simulink model "flexible_drive_filtered"  (R2022a)
settings: Solver=ode45  StartTime=0.0  StopTime=2  RelTol=1e-3  EnableMultiTasking=on
values from neighbouring files (symbols this model uses):
  b1 = 0.0097    [q1_2.m]
  b2 = 0.00097122    [q1_2.m]
  d1 = 0.793    [q1_2.m]
  d2 = 0.0793    [q1_2.m]
  k = 0.0466    [q1_2.m]
  m1 = 0.00031218    [q1_2.m]
  m2 = 0.00016858    [q1_2.m]
undefined symbols (not defined in the file or in its folder): c, kp, q, sgn, Ts
settings Model: Creator=user  LastModifiedBy=mluser
settings SolverCC: AlgebraicLoopSolver=TrustRegion
settings DataIOCC: LimitDataPoints=on  SaveFormat=Array  SignalLoggingSaveFormat=ModelDataLogs  ReturnWorkspaceOutputs=off  SignalLoggingName=sigsOut
settings OptimizationCC: LifeSpan=inf
settings DebuggingCC: SaveWithParameterizedLinksMsg=none  UnderspecifiedInitializationDetection=Classic  MergeDetectMultiDrivingBlocksExec=none  SignalResolutionControl=TryResolveAllWithWarning  MultiTaskDSMMsg=warning  MultiTaskCondExecSysMsg=none  UnconnectedInputMsg=warning  UnconnectedOutputMsg=warning  UnconnectedLineMsg=warning  SFUnexpectedBacktrackingDiag=warning  SFNoUnconditionalDefaultTransitionDiag=warning  SFMachineParentedDataDiag=warning  ArithmeticOperatorsInVariantConditions=warning
settings HardwareCC: ProdBitPerPointer=32  ProdBitPerSizeT=32  ProdBitPerPtrDiffT=32  ProdLargestAtomicFloat=None  ProdIntDivRoundTo=Undefined  ProdEndianess=Unspecified  ProdWordSize=32  ProdHWDeviceType=32-bit Generic  TargetUnknown=on
settings ModelReferenceCC: PropagateSignalLabelsOutOfModel=off
settings SFSimCC: SimUseLocalCustomCode=off  CustomCodeUndefinedFunction=UseInterfaceOnly
settings RTWCC: RTWUseLocalCustomCode=off
settings CodeAppCC: StateflowObjectComments=on
settings GRTTargetCC: TargetLangStandard=C89/C90 (ANSI)  CombineOutputUpdateFcns=off  GRTInterface=on
settings ConfigComp: CovMetricSettings=dw  CovSaveCumulativeToWorkspaceVar=on  CovSaveSingleToWorkspaceVar=on  CovExternalEMLEnable=off

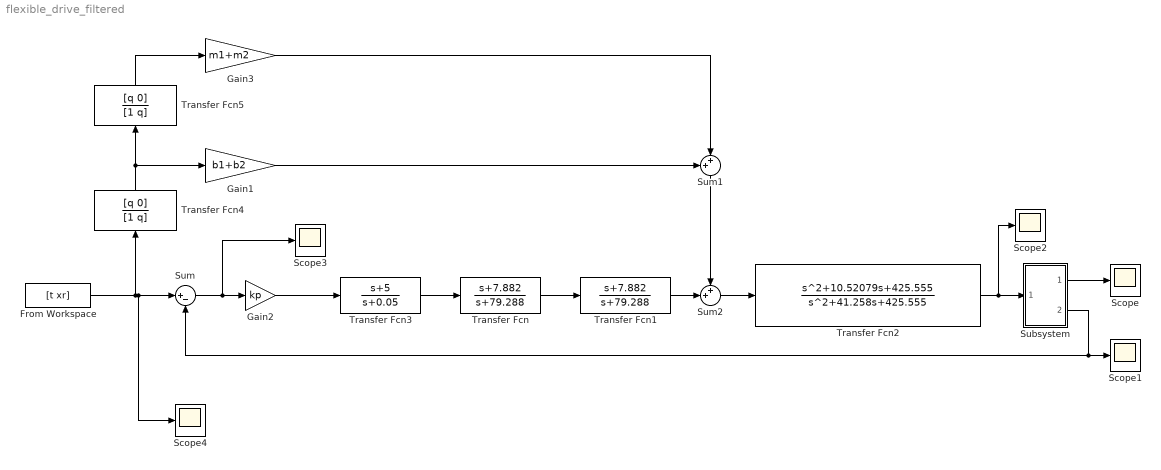
== system flexible_drive_filtered ==
  From Workspace : FromWorkspace  VariableName=[t xr]  SampleTime=Ts  ZeroCross=off  OutputAfterFinalValue=Holding final value
  Gain1 : Gain  Gain=b1+b2
  Gain2 : Gain  Gain=kp
  Gain3 : Gain  Gain=m1+m2
  Scope{,1..4} (5 alike) : Scope
  Subsystem : Subsystem
  Sum : Sum  Inputs=|+-
  Sum1 : Sum  Inputs=++|
  Sum2 : Sum  Inputs=++|
  Transfer Fcn : TransferFcn  Numerator=[1 7.882]  Denominator=[1 79.288]
  Transfer Fcn1 : TransferFcn  Numerator=[1 7.882]  Denominator=[1 79.288]
  Transfer Fcn2 : TransferFcn  Numerator=[1 10.52079 425.555]  Denominator=[1 41.258 425.555]
  Transfer Fcn3 : TransferFcn  Numerator=[1 5]  Denominator=[1 0.05]
  Transfer Fcn4 : TransferFcn  Numerator=[q 0]  Denominator=[1 q]
  Transfer Fcn5 : TransferFcn  Numerator=[q 0]  Denominator=[1 q]
  wires:
  From Workspace/1 -> Sum/1, Scope4/1, Transfer Fcn4/1
  Transfer Fcn2/1 -> Scope2/1, Subsystem/1(In1)
  Subsystem/1(Out1) -> Scope/1
  Subsystem/2(Out2) -> Scope1/1, Sum/2
  Transfer Fcn/1 -> Transfer Fcn1/1
  Sum/1 -> Scope3/1, Gain2/1
  Gain2/1 -> Transfer Fcn3/1
  Transfer Fcn3/1 -> Transfer Fcn/1
  Transfer Fcn4/1 -> Gain1/1, Transfer Fcn5/1
  Transfer Fcn5/1 -> Gain3/1
  Sum2/1 -> Transfer Fcn2/1
  Gain3/1 -> Sum1/2
  Gain1/1 -> Sum1/1
  Transfer Fcn1/1 -> Sum2/2
  Sum1/1 -> Sum2/1

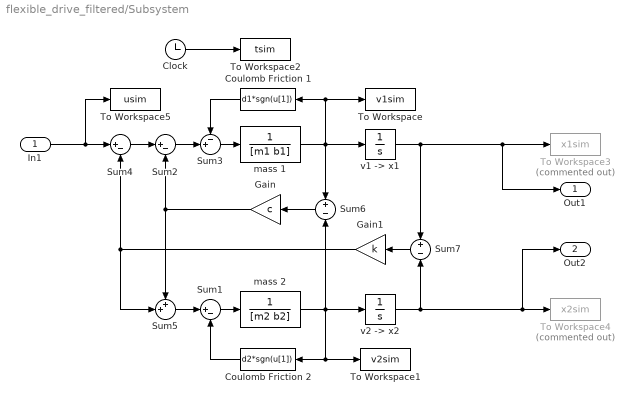
== system flexible_drive_filtered/Subsystem ==
  In1 : Inport
  Clock : Clock
  Coulomb Friction 1 : Fcn  Expr=d1*sgn(u[1])
  Coulomb Friction 2 : Fcn  Expr=d2*sgn(u[1])
  Gain : Gain  Gain=c  SaturateOnIntegerOverflow=on  OutDataTypeStr=Inherit: Same as input  ParamDataTypeStr=Inherit: Same as input
  Gain1 : Gain  Gain=k  SaturateOnIntegerOverflow=on  OutDataTypeStr=Inherit: Same as input  ParamDataTypeStr=Inherit: Same as input
  Sum1 : Sum  Inputs=|+-  SaturateOnIntegerOverflow=on
  Sum2 : Sum  Inputs=|+-  SaturateOnIntegerOverflow=on
  Sum3 : Sum  Inputs=-+|  SaturateOnIntegerOverflow=on
  Sum4 : Sum  Inputs=|+-  SaturateOnIntegerOverflow=on
  Sum5 : Sum  Inputs=++|  SaturateOnIntegerOverflow=on
  Sum6 : Sum  Inputs=+|-  SaturateOnIntegerOverflow=on
  Sum7 : Sum  Inputs=+|-  SaturateOnIntegerOverflow=on
  To Workspace : ToWorkspace  VariableName=v1sim  SampleTime=Ts
  To Workspace1 : ToWorkspace  VariableName=v2sim  SampleTime=Ts
  To Workspace2 : ToWorkspace  VariableName=tsim  SampleTime=Ts
  To Workspace3 : ToWorkspace  Commented=on  VariableName=x1sim  SampleTime=Ts
  To Workspace4 : ToWorkspace  Commented=on  VariableName=x2sim  SampleTime=Ts
  To Workspace5 : ToWorkspace  VariableName=usim  SampleTime=Ts
  mass 1 : TransferFcn  Denominator=[m1 b1]
  mass 2 : TransferFcn  Denominator=[m2 b2]
  "v1 -> x1" : Integrator
  "v2 -> x2" : Integrator
  Out1 : Outport
  Out2 : Outport  Port=2
  wires:
  Coulomb Friction 1/1 -> Sum3/1
  In1/1 -> Sum4/1, To Workspace5/1
  Coulomb Friction 2/1 -> Sum1/2
  Sum4/1 -> Sum2/1
  Sum5/1 -> Sum1/1
  Sum2/1 -> Sum3/2
  Sum6/1 -> Gain/1
  Sum1/1 -> mass 2/1
  Sum7/1 -> Gain1/1
  Gain/1 -> Sum2/2, Sum5/1
  Gain1/1 -> Sum4/2, Sum5/2
  Clock/1 -> To Workspace2/1
  mass 1/1 -> "v1 -> x1"/1, Sum6/1, Coulomb Friction 1/1, To Workspace/1
  mass 2/1 -> "v2 -> x2"/1, Sum6/2, Coulomb Friction 2/1, To Workspace1/1
  "v1 -> x1"/1 -> Sum7/1, Out1/1, To Workspace3/1
  "v2 -> x2"/1 -> Sum7/2, Out2/1, To Workspace4/1
  Sum3/1 -> mass 1/1
